simulink model "Passive_Cell_Balancing_Method"  (R2022a)
settings: Solver=VariableStepAuto  StartTime=0.0  StopTime=10.0  RelTol=1e-3
undefined symbols (not defined in the file or in its folder): Ion, Lithium
libraries: spsBatteryLib x3, spsIdealSwitchLib x3, spsSeriesRLCLoadLib x3, spspowerguiLib x1
settings Model: Creator=nikos  LastModifiedBy=nikos

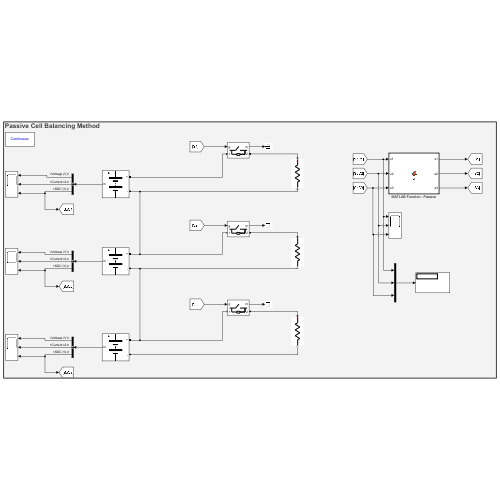
[thumbnail: Simulink's stored preview of the top-level diagram]
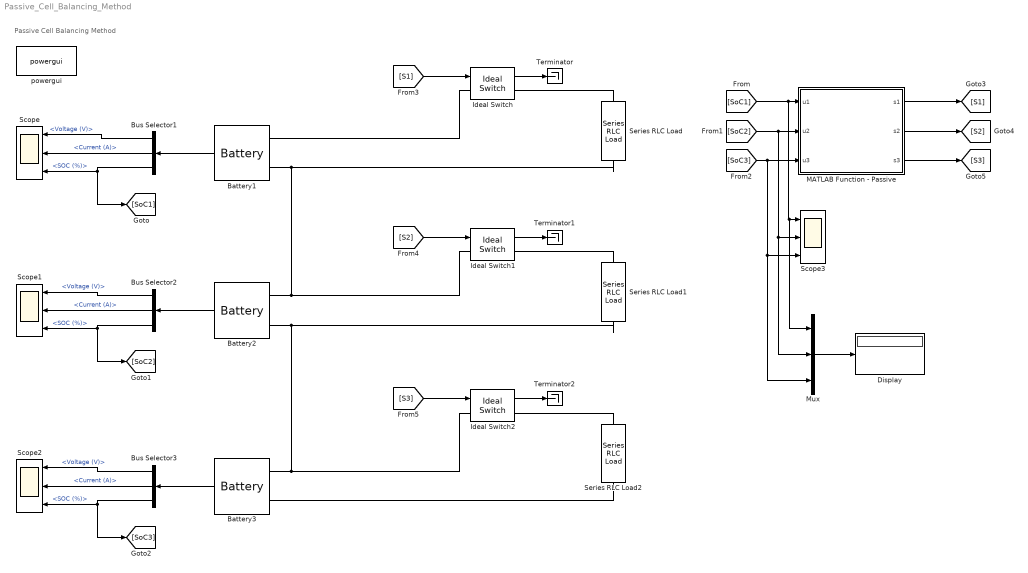
== system Passive_Cell_Balancing_Method ==
  note: Passive Cell Balancing Method
  Battery1 : spsBatteryLib/Battery  BatType=Lithium-Ion  ShowTempParam=off  ThermalPreset=no  ShowAgeParam=off  NomV=3.7  NomQ=4  SOC=60  Batt_Tr=1  PresetModel=on  MaxQ=4  MinV=2.775  FullV=4.3068  Dis_rate=1.7391  R=0.00925  Normal_OP=3.6174  expZone="[3.9974     0.19652]"  current=[6.5 13 32.5]  Units=Time  Tci=20  NomT=20  T2=-30  MaxQ2=4.8  FullV2=7.1  Normal_OP2=5.655  expZone2="[6.58           1]"  Rca=0.6  ti=2000  Dp=0  Neq0=0  Tsim=1e6  Ta1=25  Qeol=5.4*0.9  Reol=0.013333*1.2  Char_age=[2.3478, 3]  Dis_age=[2.3478, 10]  N1=1500  N2=10500  N3=1000  N4=1400  Ta2=45  N5=950
  Battery2 : spsBatteryLib/Battery  BatType=Lithium-Ion  ShowTempParam=off  ThermalPreset=no  ShowAgeParam=off  NomV=3.7  NomQ=4  SOC=40  Batt_Tr=1  PresetModel=on  MaxQ=4  MinV=2.775  FullV=4.3068  Dis_rate=1.7391  R=0.00925  Normal_OP=3.6174  expZone="[3.9974     0.19652]"  current=[6.5 13 32.5]  Units=Time  Tci=20  NomT=20  T2=-30  MaxQ2=4.8  FullV2=7.1  Normal_OP2=5.655  expZone2="[6.58           1]"  Rca=0.6  ti=2000  Dp=0  Neq0=0  Tsim=1e6  Ta1=25  Qeol=5.4*0.9  Reol=0.013333*1.2  Char_age=[2.3478, 3]  Dis_age=[2.3478, 10]  N1=1500  N2=10500  N3=1000  N4=1400  Ta2=45  N5=950
  Battery3 : spsBatteryLib/Battery  BatType=Lithium-Ion  ShowTempParam=off  ThermalPreset=no  ShowAgeParam=off  NomV=3.7  NomQ=4  SOC=35  Batt_Tr=1  PresetModel=on  MaxQ=4  MinV=2.775  FullV=4.3068  Dis_rate=1.7391  R=0.00925  Normal_OP=3.6174  expZone="[3.9974     0.19652]"  current=[6.5 13 32.5]  Units=Time  Tci=20  NomT=20  T2=-30  MaxQ2=4.8  FullV2=7.1  Normal_OP2=5.655  expZone2="[6.58           1]"  Rca=0.6  ti=2000  Dp=0  Neq0=0  Tsim=1e6  Ta1=25  Qeol=5.4*0.9  Reol=0.013333*1.2  Char_age=[2.3478, 3]  Dis_age=[2.3478, 10]  N1=1500  N2=10500  N3=1000  N4=1400  Ta2=45  N5=950
  Bus Selector1 : BusSelector  OutputSignals=Voltage (V),Current (A),SOC (%)
  Bus Selector2 : BusSelector  OutputSignals=Voltage (V),Current (A),SOC (%)
  Bus Selector3 : BusSelector  OutputSignals=Voltage (V),Current (A),SOC (%)
  Display : Display
  Ideal Switch : spsIdealSwitchLib/Ideal Switch  Ron=0.001  Lon=0  IC=0  Rs=1e5  Cs=inf  Measurements=on
  Ideal Switch1 : spsIdealSwitchLib/Ideal Switch  Ron=0.001  Lon=0  IC=0  Rs=1e5  Cs=inf  Measurements=on
  Ideal Switch2 : spsIdealSwitchLib/Ideal Switch  Ron=0.001  Lon=0  IC=0  Rs=1e5  Cs=inf  Measurements=on
  MATLAB Function - Passive : MATLAB Function  TreatAsAtomicUnit=on
  Mux : Mux  Inputs=3
  Scope{,1..3} (4 alike) : Scope  NumInputPorts=3
  Series RLC Load : spsSeriesRLCLoadLib/Series RLC Load  LConnTagsString=a  RConnTagsString=__new0  NominalVoltage=4  NominalFrequency=0.1  ActivePower=1e3  InductivePower=0  CapacitivePower=0  Setx0=off  InitialVoltage=0  SetiL0=off  InitialCurrent=0  Measurements=None  LoadType=constant Z
  Series RLC Load1 : spsSeriesRLCLoadLib/Series RLC Load  LConnTagsString=a  RConnTagsString=__new0  NominalVoltage=4  NominalFrequency=0.1  ActivePower=1e3  InductivePower=0  CapacitivePower=0  Setx0=off  InitialVoltage=0  SetiL0=off  InitialCurrent=0  Measurements=None  LoadType=constant Z
  Series RLC Load2 : spsSeriesRLCLoadLib/Series RLC Load  LConnTagsString=a  RConnTagsString=__new0  NominalVoltage=4  NominalFrequency=0.1  ActivePower=1e3  InductivePower=0  CapacitivePower=0  Setx0=off  InitialVoltage=0  SetiL0=off  InitialCurrent=0  Measurements=None  LoadType=constant Z
  Terminator : Terminator
  Terminator1 : Terminator
  Terminator2 : Terminator
  powergui : spspowerguiLib/powergui  Priority=1  SimulationMode=Continuous  SampleTime=50e-6  frequency=60  Iterations=50  frequencyindice=0  Pbase=100e6  ErrMax=1e-4  UnitsV=kV  UnitsW=MW  buscounter=0  FunctionMessages=off  echomessages=off  EnableUseOfTLC=off  CurrentSourceSwitches=off  DisableSnubberDevices=off  DisableRonSwitches=off  DisableVfSwitches=off  DisplayEquations=off  AutomaticDiscreteSolvers=off  SolverType=Tustin/Backward Euler (TBE)  Interpol=off  ExternalGateDelay=off  methode=off  Ts=100  x0status=blocks  SPID=on  SwTol=0  HookPort=off  NonlinearTolerance=1e-4  nMaxIteration=100  ContinueOnMaxIteration=off  RestoreLinks=warning  ResistiveCurrentMeasurement=off  Frange=[0:2:500]  Ylog=off  Xlog=on  ShowGrid=off  save=off  variable=ZData  structure=0  ZoomFFT=off  StartTime=0.0  cycles=1  DisplayStyle=1  fundamental=60  FreqAxis=off  MaxFrequency=1000  frequencyindicesteady=1  RmsSteady=1  display=off
  wires:
  Bus Selector1/1 -> Scope/1  "<Voltage (V)>"
  [SoC1] -> Mux/1, Scope3/1, MATLAB Function - Passive/1(u1)
  MATLAB Function - Passive/2(s2) -> [S2]
  Bus Selector2/3 -> [SoC2], Scope1/3  "<SOC (%)>"
  Battery2/1 -> Bus Selector2/1
  Bus Selector3/1 -> Scope2/1  "<Voltage (V)>"
  Battery1/1 -> Bus Selector1/1
  [S2] -> Ideal Switch1/1
  Bus Selector2/1 -> Scope1/1  "<Voltage (V)>"
  [S3] -> Ideal Switch2/1
  [S1] -> Ideal Switch/1
  Ideal Switch2/1 -> Terminator2/1
  Mux/1 -> Display/1
  Battery3/1 -> Bus Selector3/1
  Ideal Switch1/1 -> Terminator1/1
  Bus Selector3/3 -> [SoC3], Scope2/3  "<SOC (%)>"
  Bus Selector3/2 -> Scope2/2  "<Current (A)>"
  Ideal Switch/1 -> Terminator/1
  Bus Selector2/2 -> Scope1/2  "<Current (A)>"
  [SoC3] -> Mux/3, Scope3/3, MATLAB Function - Passive/3(u3)
  Bus Selector1/3 -> [SoC1], Scope/3  "<SOC (%)>"
  [SoC2] -> Mux/2, Scope3/2, MATLAB Function - Passive/2(u2)
  MATLAB Function - Passive/3(s3) -> [S3]
  MATLAB Function - Passive/1(s1) -> [S1]
  Bus Selector1/2 -> Scope/2  "<Current (A)>"
  connections:
  Battery3/LConn1 -- Ideal Switch2/LConn1 -- Series RLC Load1/RConn1 -- Battery2/LConn2
  Series RLC Load/RConn1 -- Battery1/LConn2 -- Battery2/LConn1 -- Ideal Switch1/LConn1
  Series RLC Load2/RConn1 -- Battery3/LConn2
  Series RLC Load/LConn1 -- Ideal Switch/RConn1
  Ideal Switch/LConn1 -- Battery1/LConn1
  Series RLC Load1/LConn1 -- Ideal Switch1/RConn1
  Series RLC Load2/LConn1 -- Ideal Switch2/RConn1

== matlab function Passive_Cell_Balancing_Method/MATLAB Function - Passive ==
  data: u1 input; s1 output; u2 input; u3 input; s2 output; s3 output
function [s1, s2, s3] = fcn(u1, u2, u3)

u1 = int32(u1);
u2 = int32(u2);
u3 = int32(u3);

if ((u1 > u2) || (u1> u3))
    s1 = 1;
else 
    s1 = 0;
end

if ((u2 > u1) || (u2 > u3))
    s2 = 1;
else
    s2 = 0;
end

if ((u3 > u1) || (u3 > u2))
    s3 = 1;
else
    s3 = 0;
end
